simulink model "PGEReducedOrderModel"  (Simulink 8.7)
settings: Solver=ode23tb  StartTime=0.0  StopTime=4  MaxStep=0.04  RelTol=1e-3
undefined symbols (not defined in the file): D1, Delta
libraries: powerlib x98
Description:
  | Copyright 2008-2016 The MathWorks, Inc.
settings Model: Creator=MathWorks  LastModifiedBy=Sayonsom Chanda
settings DataIOCC: SignalLoggingSaveFormat=ModelDataLogs
settings OptimizationCC: ExpressionDepthLimit=2147483647
settings DebuggingCC: SolverPrmCheckMsg=warning  FcnCallInpInsideContextMsg=UseLocalSettings  UnconnectedInputMsg=none  UnconnectedOutputMsg=none  UnconnectedLineMsg=none  StateNameClashWarn=warning
settings GRTTargetCC: CombineOutputUpdateFcns=off  GRTInterface=on
settings ConfigComp: CovSFcnEnable=off

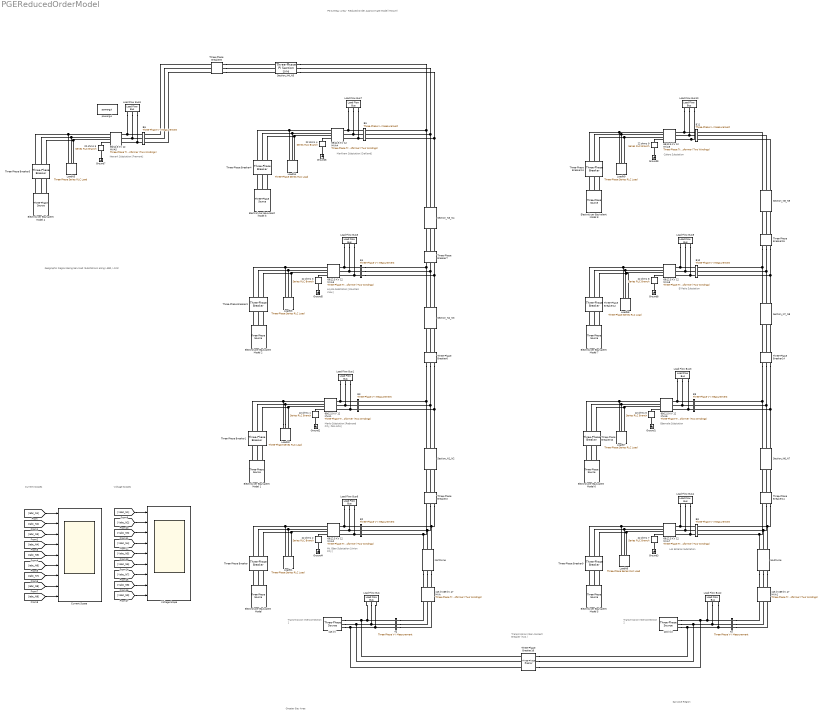
== system PGEReducedOrderModel ==
  note: Geographic Region Being Serviced
      | (Substations along I-880, I-101)
  note: Mt. Eden
      | Substation
      | [Union City]
  note: PG & E Bay Area - Reduced Order Approximate Model (ROAM)
  note: Transmission
      | Interconnection 1
  note: Menlo
      | Substation
      | [Redwood City,
      | Palo Alto]
  note: Loyola
      | Substation
      | [Mountain View]
  note: Markham
      | Substation
      | [Oakland]
  note: Newark
      | Substation
      | [Fremont]
  note: Los Esteros
      | Substation
  note: Transmission
      | Interconnection 2
  note: Edenvale
      | Substation
  note: Calero
      | Substation
  note: Transmission
      | Inter-connect
      | Breaker (N.O.)
  note: Greater Bay Area
  note: San Jose Region
  note: El Patio
      | Substation
  note: Voltage Scopes
  note: Current Scopes
  115 kV : powerlib/Electrical Sources/Three-Phase Source  InternalConnection=Yg  VoltagePhases=off  Voltage=(115000)*1.0445  PhaseAngle=-3.3182  Voltage_phases=[25e3 25e3 25e3]/sqrt(3)  PhaseAngles_phases=[0 -120 +120]  Frequency=60  NonIdealSource=on  SpecifyImpedance=on  Resistance=0.8929  Inductance=16.58e-3  ShortCircuitLevel=2000e6  BaseVoltage=120e3  XRratio=7  BusType=swing  Pref=10000000  Qref=3000000  Prefabc=[10e3, 10e3, 10e3]  Qrefabc=[0, 0, 0]  Qmin=-Inf  Qmax=Inf
  115 kV/69 kV 47 MVA : powerlib/Elements/Three-Phase Transformer (Two Windings)  Winding1Connection=Yg  Winding2Connection=Delta (D1)  CoreType=Three single-phase transformers  SetSaturation=off  Hysteresis=off  DataFile='basic_model'  SetInitialFlux=off  Measurements=None  UNITS=pu  NominalPower=[47e6 60 ]  Winding1="[ 115e3  0.002    0.06 ]"  Winding2="[ 69e3  0.002  0.06]"  Rm=500  Lm=500  L0=0.5  Saturation="[ 0,0  ;  0.005,1.2  ;  1.0,1.4 ]"  InitialFluxes=[ 0.8 , -0.8 , 0.7 ]  MoreParameters=off  BreakLoop=off  DataType=off  TransfoNumber=0
  115 kV/69 kV 47 MVA1 : powerlib/Elements/Three-Phase Transformer (Two Windings)  Winding1Connection=Yg  Winding2Connection=Delta (D1)  CoreType=Three single-phase transformers  SetSaturation=off  Hysteresis=off  DataFile='basic_model'  SetInitialFlux=off  Measurements=None  UNITS=pu  NominalPower=[47e6 60 ]  Winding1="[ 115e3  0.002    0.06 ]"  Winding2="[ 69e3  0.002  0.06]"  Rm=500  Lm=500  L0=0.5  Saturation="[ 0,0  ;  0.005,1.2  ;  1.0,1.4 ]"  InitialFluxes=[ 0.8 , -0.8 , 0.7 ]  MoreParameters=off  BreakLoop=off  DataType=off  TransfoNumber=0
  115 kV2 : powerlib/Electrical Sources/Three-Phase Source  InternalConnection=Yg  VoltagePhases=off  Voltage=(115000)*1.0445  PhaseAngle=-3.3182  Voltage_phases=[25e3 25e3 25e3]/sqrt(3)  PhaseAngles_phases=[0 -120 +120]  Frequency=60  NonIdealSource=on  SpecifyImpedance=on  Resistance=0.8929  Inductance=16.58e-3  ShortCircuitLevel=2000e6  BaseVoltage=115e3  XRratio=7  BusType=swing  Pref=10000000  Qref=3000000  Prefabc=[10e3, 10e3, 10e3]  Qrefabc=[0, 0, 0]  Qmin=-Inf  Qmax=Inf
  22 ohms {1..9} (9 alike) : powerlib/Elements/Series RLC Branch  LConnTagsString=__new0  RConnTagsString=__new0  BranchType=R  Resistance=22  Inductance=1.0  SetiL0=off  InitialCurrent=0  Capacitance=1.0  Setx0=off  InitialVoltage=0  Measurements=None
  69/12.5 KV 12 MVA{1..9} (9 alike) : powerlib/Elements/Three-Phase Transformer (Two Windings)  Winding1Connection=Yg  Winding2Connection=Yn  CoreType=Three single-phase transformers  SetSaturation=off  Hysteresis=off  DataFile='hysteresis'  SetInitialFlux=off  Measurements=None  UNITS=pu  NominalPower="[12e6  60]"  Winding1=[69e3 , 0.025/30 , 0.025]  Winding2=[ 12500, 0.025/30 , 0.025]  Rm=500  Lm=inf  L0=0.5  Saturation=[ 0,0 ; 0.0024,1.2 ; 1.0,1.52 ]  InitialFluxes=[ 0.8 , -0.8 , 0.7 ]  MoreParameters=off  BreakLoop=off  DataType=off  TransfoNumber=0
  B10 : powerlib/Measurements/Three-Phase V-I Measurement  VoltageMeasurement=phase-to-ground  SetLabelV=on  LabelV=Vabc_N8  Vpu=on  VpuLL=off  CurrentMeasurement=yes  SetLabelI=on  LabelI=Iabc_N8  Ipu=on  Pbase=10e6  Vbase=69e3  OutputType=Complex  PhasorSimulation=on  PSBequivalent=0
  B11 : powerlib/Measurements/Three-Phase V-I Measurement  VoltageMeasurement=phase-to-ground  SetLabelV=on  LabelV=Vabc_N9  Vpu=on  VpuLL=off  CurrentMeasurement=yes  SetLabelI=on  LabelI=Iabc_N9  Ipu=on  Pbase=10e6  Vbase=69e3  OutputType=Complex  PhasorSimulation=on  PSBequivalent=0
  B2 : powerlib/Measurements/Three-Phase V-I Measurement  VoltageMeasurement=phase-to-ground  SetLabelV=on  LabelV=Vabc_N1  Vpu=on  VpuLL=off  CurrentMeasurement=yes  SetLabelI=on  LabelI=Iabc_N1  Ipu=on  Pbase=10e6  Vbase=69e3  OutputType=Complex  PhasorSimulation=on  PSBequivalent=0
  B3 : powerlib/Measurements/Three-Phase V-I Measurement  VoltageMeasurement=phase-to-ground  SetLabelV=on  LabelV=Vabc_N2  Vpu=on  VpuLL=off  CurrentMeasurement=yes  SetLabelI=on  LabelI=Iabc_N2  Ipu=on  Pbase=10e6  Vbase=69e3  OutputType=Complex  PhasorSimulation=on  PSBequivalent=0
  B4 : powerlib/Measurements/Three-Phase V-I Measurement  VoltageMeasurement=phase-to-ground  SetLabelV=on  LabelV=Vabc_N3  Vpu=on  VpuLL=off  CurrentMeasurement=yes  SetLabelI=on  LabelI=Iabc_N3  Ipu=on  Pbase=10e6  Vbase=69e3  OutputType=Complex  PhasorSimulation=on  PSBequivalent=0
  B5 : powerlib/Measurements/Three-Phase V-I Measurement  VoltageMeasurement=phase-to-ground  SetLabelV=on  LabelV=Vabc_N4  Vpu=on  VpuLL=off  CurrentMeasurement=yes  SetLabelI=on  LabelI=Iabc_N4  Ipu=on  Pbase=10e6  Vbase=69e3  OutputType=Complex  PhasorSimulation=on  PSBequivalent=0
  B6 : powerlib/Measurements/Three-Phase V-I Measurement  VoltageMeasurement=phase-to-ground  SetLabelV=on  LabelV=Vabc_N5  Vpu=on  VpuLL=off  CurrentMeasurement=yes  SetLabelI=on  LabelI=Iabc_N5  Ipu=on  Pbase=10e6  Vbase=69e3  OutputType=Complex  PhasorSimulation=on  PSBequivalent=0
  B8 : powerlib/Measurements/Three-Phase V-I Measurement  VoltageMeasurement=phase-to-ground  SetLabelV=on  LabelV=Vabc_N6  Vpu=on  VpuLL=off  CurrentMeasurement=yes  SetLabelI=on  LabelI=Iabc_N6  Ipu=on  Pbase=10e6  Vbase=12.5e3  OutputType=Complex  PhasorSimulation=on  PSBequivalent=0
  B9 : powerlib/Measurements/Three-Phase V-I Measurement  VoltageMeasurement=phase-to-ground  SetLabelV=on  LabelV=Vabc_N7  Vpu=on  VpuLL=off  CurrentMeasurement=yes  SetLabelI=on  LabelI=Iabc_N7  Ipu=on  Pbase=10e6  Vbase=69e3  OutputType=Complex  PhasorSimulation=on  PSBequivalent=0
  Current Scope : Scope  NumInputPorts=9
  Electrolyzer Equivalent Model {,2..8} (8 alike) : powerlib/Electrical Sources/Three-Phase Source  InternalConnection=Yg  VoltagePhases=off  Voltage=12.5e3  PhaseAngle=0  Voltage_phases=[25e3 25e3 25e3]/sqrt(3)  PhaseAngles_phases=[0 -120 +120]  Frequency=60  NonIdealSource=on  SpecifyImpedance=off  Resistance=0.8929  Inductance=16.58e-3  ShortCircuitLevel=100e6  BaseVoltage=25e3  XRratio=7  BusType=PQ  Pref=10e3  Qref=0  Prefabc=[10e3, 10e3, 10e3]  Qrefabc=[0, 0, 0]  Qmin=-inf  Qmax=inf
  Electrolyzer Equivalent Model 1 : powerlib/Electrical Sources/Three-Phase Source  InternalConnection=Yg  VoltagePhases=off  Voltage=12.5e3  PhaseAngle=0  Voltage_phases=[25e3 25e3 25e3]/sqrt(3)  PhaseAngles_phases=[0 -120 +120]  Frequency=60  NonIdealSource=on  SpecifyImpedance=off  Resistance=0.8929  Inductance=16.58e-3  ShortCircuitLevel=100e6  BaseVoltage=12.5e3  XRratio=7  BusType=PQ  Pref=10e3  Qref=0  Prefabc=[10e3, 10e3, 10e3]  Qrefabc=[0, 0, 0]  Qmin=-inf  Qmax=inf
  Ground{1..9} (9 alike) : powerlib/Elements/Ground  LConnTagsString=a
  Load Flow Bus : powerlib/Measurements/Load Flow Bus  LConnTagsString=a|b|c  Phases=ABC  Connectors=on one side  ID=T1  Vbase=115e3  Vref=1.02  Vangle=0  VLF=1.02  VLFb=1  VLFc=1  angleLF=0  angleLFb=0  angleLFc=0
      settings: AttributesFormatString=%<ID>\n%<Vbase>V\n%<VLF>pu\n%<angleLF>deg.
  Load Flow Bus1 : powerlib/Measurements/Load Flow Bus  LConnTagsString=a|b|c  Phases=ABC  Connectors=on one side  ID=N2  Vbase=69e3  Vref=1.02  Vangle=0  VLF=1.02  VLFb=1  VLFc=1  angleLF=0  angleLFb=0  angleLFc=0
      settings: AttributesFormatString=%<ID>\n%<Vbase>V\n%<VLF>pu\n%<angleLF>deg.
  Load Flow Bus10 : powerlib/Measurements/Load Flow Bus  LConnTagsString=a|b|c  Phases=ABC  Connectors=on one side  ID=N9  Vbase=69e3  Vref=1.02  Vangle=0  VLF=1.02  VLFb=1  VLFc=1  angleLF=0  angleLFb=0  angleLFc=0
      settings: AttributesFormatString=%<ID>\n%<Vbase>V\n%<VLF>pu\n%<angleLF>deg.
  Load Flow Bus2 : powerlib/Measurements/Load Flow Bus  LConnTagsString=a|b|c  Phases=ABC  Connectors=on one side  ID=T2  Vbase=115e3  Vref=1.02  Vangle=0  VLF=1.02  VLFb=1  VLFc=1  angleLF=0  angleLFb=0  angleLFc=0
      settings: AttributesFormatString=%<ID>\n%<Vbase>V\n%<VLF>pu\n%<angleLF>deg.
  Load Flow Bus3 : powerlib/Measurements/Load Flow Bus  LConnTagsString=a|b|c  Phases=ABC  Connectors=on one side  ID=N7  Vbase=69e3  Vref=1.02  Vangle=0  VLF=1.02  VLFb=1  VLFc=1  angleLF=0  angleLFb=0  angleLFc=0
      settings: AttributesFormatString=%<ID>\n%<Vbase>V\n%<VLF>pu\n%<angleLF>deg.
  Load Flow Bus4 : powerlib/Measurements/Load Flow Bus  LConnTagsString=a|b|c  Phases=ABC  Connectors=on one side  ID=N6  Vbase=69e3  Vref=1.02  Vangle=0  VLF=1.02  VLFb=1  VLFc=1  angleLF=0  angleLFb=0  angleLFc=0
      settings: AttributesFormatString=%<ID>\n%<Vbase>V\n%<VLF>pu\n%<angleLF>deg.
  Load Flow Bus5 : powerlib/Measurements/Load Flow Bus  LConnTagsString=a|b|c  Phases=ABC  Connectors=on one side  ID=N3  Vbase=69e3  Vref=1.02  Vangle=0  VLF=1.02  VLFb=1  VLFc=1  angleLF=0  angleLFb=0  angleLFc=0
      settings: AttributesFormatString=%<ID>\n%<Vbase>V\n%<VLF>pu\n%<angleLF>deg.
  Load Flow Bus6 : powerlib/Measurements/Load Flow Bus  LConnTagsString=a|b|c  Phases=ABC  Connectors=on one side  ID=N1  Vbase=69e3  Vref=1.02  Vangle=0  VLF=1.02  VLFb=1  VLFc=1  angleLF=0  angleLFb=0  angleLFc=0
      settings: AttributesFormatString=%<ID>\n%<Vbase>V\n%<VLF>pu\n%<angleLF>deg.
  Load Flow Bus7 : powerlib/Measurements/Load Flow Bus  LConnTagsString=a|b|c  Phases=ABC  Connectors=on one side  ID=N4  Vbase=69e3  Vref=1.02  Vangle=0  VLF=1.02  VLFb=1  VLFc=1  angleLF=0  angleLFb=0  angleLFc=0
      settings: AttributesFormatString=%<ID>\n%<Vbase>V\n%<VLF>pu\n%<angleLF>deg.
  Load Flow Bus8 : powerlib/Measurements/Load Flow Bus  LConnTagsString=a|b|c  Phases=ABC  Connectors=on one side  ID=N5  Vbase=69e3  Vref=1.02  Vangle=0  VLF=1.02  VLFb=1  VLFc=1  angleLF=0  angleLFb=0  angleLFc=0
      settings: AttributesFormatString=%<ID>\n%<Vbase>V\n%<VLF>pu\n%<angleLF>deg.
  Load Flow Bus9 : powerlib/Measurements/Load Flow Bus  LConnTagsString=a|b|c  Phases=ABC  Connectors=on one side  ID=N8  Vbase=69e3  Vref=1.02  Vangle=0  VLF=1.02  VLFb=1  VLFc=1  angleLF=0  angleLFb=0  angleLFc=0
      settings: AttributesFormatString=%<ID>\n%<Vbase>V\n%<VLF>pu\n%<angleLF>deg.
  LoadN1 : powerlib/Elements/Three-Phase Series RLC Load  LConnTagsString=A|B|C  Configuration=Delta  NominalVoltage=12.5e3  Vabc=[1e3 1e3 1e3]  Vabcp=[1e3 1e3 1e3]  NominalFrequency=60  UnbalancedPower=off  ActivePower=0.89e6/50  InductivePower=0  CapacitivePower=1.2e6  Pabc=[10e3 9e3 11e3]  QLabc=[100 90 110]  QCabc=[100 90 110]  Pabcp=[10e3 9e3 11e3]  QLabcp=[100 90 110]  QCabcp=[100 90 110]  Measurements=None  LoadType=constant PQ
  LoadN{2..9} (8 alike) : powerlib/Elements/Three-Phase Series RLC Load  LConnTagsString=A|B|C  Configuration=Delta  NominalVoltage=12.5e3  Vabc=[1e3 1e3 1e3]  Vabcp=[1e3 1e3 1e3]  NominalFrequency=60  UnbalancedPower=off  ActivePower=1.2e6/50  InductivePower=0  CapacitivePower=1.2e6  Pabc=[10e3 9e3 11e3]  QLabc=[100 90 110]  QCabc=[100 90 110]  Pabcp=[10e3 9e3 11e3]  QLabcp=[100 90 110]  QCabcp=[100 90 110]  Measurements=None  LoadType=constant PQ
  NorthLine : powerlib/Elements/Three-Phase PI Section Line  LConnTagsString=a|b|c  RConnTagsString=A|B|C  Frequency=60  Resistances=[0.1153 0.413]  Inductances=[1.05e-3 3.32e-3]  Capacitances=[11.33e-009 5.01e-009]  Length=25
  Section_N1_N2 : powerlib/Elements/Three-Phase PI Section Line  LConnTagsString=a|b|c  RConnTagsString=A|B|C  Frequency=60  Resistances=[0.1153 0.413]  Inductances=[1.05e-3 3.32e-3]  Capacitances=[11.33e-009 5.01e-009]  Length=25
  Section_N2_N3 : powerlib/Elements/Three-Phase PI Section Line  LConnTagsString=a|b|c  RConnTagsString=A|B|C  Frequency=60  Resistances=[0.1153 0.413]  Inductances=[1.05e-3 3.32e-3]  Capacitances=[11.33e-009 5.01e-009]  Length=25
  Section_N3_N4 : powerlib/Elements/Three-Phase PI Section Line  LConnTagsString=a|b|c  RConnTagsString=A|B|C  Frequency=60  Resistances=[0.1153 0.413]  Inductances=[1.05e-3 3.32e-3]  Capacitances=[11.33e-009 5.01e-009]  Length=25
  Section_N4_N5 : powerlib/Elements/Three-Phase PI Section Line  LConnTagsString=a|b|c  RConnTagsString=A|B|C  Frequency=60  Resistances=[0.1153 0.413]  Inductances=[1.05e-3 3.32e-3]  Capacitances=[11.33e-009 5.01e-009]  Length=25
  Section_N6_N7 : powerlib/Elements/Three-Phase PI Section Line  LConnTagsString=a|b|c  RConnTagsString=A|B|C  Frequency=60  Resistances=[0.1153 0.413]  Inductances=[1.05e-3 3.32e-3]  Capacitances=[11.33e-009 5.01e-009]  Length=25
  Section_N7_N8 : powerlib/Elements/Three-Phase PI Section Line  LConnTagsString=a|b|c  RConnTagsString=A|B|C  Frequency=60  Resistances=[0.1153 0.413]  Inductances=[1.05e-3 3.32e-3]  Capacitances=[11.33e-009 5.01e-009]  Length=25
  Section_N8_N9 : powerlib/Elements/Three-Phase PI Section Line  LConnTagsString=a|b|c  RConnTagsString=A|B|C  Frequency=60  Resistances=[0.1153 0.413]  Inductances=[1.05e-3 3.32e-3]  Capacitances=[11.33e-009 5.01e-009]  Length=25
  SouthLine : powerlib/Elements/Three-Phase PI Section Line  LConnTagsString=a|b|c  RConnTagsString=A|B|C  Frequency=60  Resistances=[0.0153 0.413]  Inductances=[1.05e-3 3.32e-3]  Capacitances=[11.33e-009 5.01e-009]  Length=25
  "T1 " : powerlib/Measurements/Three-Phase V-I Measurement  VoltageMeasurement=phase-to-ground  SetLabelV=on  LabelV=T1  Vpu=on  VpuLL=off  CurrentMeasurement=no  SetLabelI=on  LabelI=Iabc_B120  Ipu=off  Pbase=100e6  Vbase=115e3  OutputType=Complex  PhasorSimulation=on  PSBequivalent=0
  "T2 " : powerlib/Measurements/Three-Phase V-I Measurement  VoltageMeasurement=phase-to-ground  SetLabelV=on  LabelV=T2  Vpu=on  VpuLL=off  CurrentMeasurement=no  SetLabelI=on  LabelI=Iabc_B120  Ipu=off  Pbase=100e6  Vbase=115e3  OutputType=Complex  PhasorSimulation=on  PSBequivalent=0
  Three-Phase Breaker{,1,3..5,9..10,12..13,16} (10 alike) : powerlib/Elements/Three-Phase Breaker  InitialState=open  SwitchA=on  SwitchB=on  SwitchC=on  SwitchTimes="[1/60  5/60]"  External=off  BreakerResistance=0.01  SnubberResistance=1e6  SnubberCapacitance=inf  Measurements=Breaker voltages
  Three-Phase Breaker{2,6..8,11,14..15} (7 alike) : powerlib/Elements/Three-Phase Breaker  InitialState=closed  SwitchA=on  SwitchB=on  SwitchC=on  SwitchTimes="[1/60  5/60]"  External=off  BreakerResistance=0.01  SnubberResistance=1e6  SnubberCapacitance=inf  Measurements=None
  Voltage Scope : Scope  NumInputPorts=9
  powergui : powerlib/powergui  Priority=1  SimulationMode=Phasor  SolverType=Tustin  SampleTime=50e-6  frequency=60  SPID=off  DisableSnubberDevices=off  DisableRonSwitches=off  DisableVfSwitches=off  SwTol=0  DisplayEquations=off  Interpol=off  ExternalGateDelay=off  methode=off  Ts=100  FunctionMessages=off  echomessages=off  HookPort=off  EnableUseOfTLC=off  x0status=blocks  frequencyindice=60  Pbase=100e6  ErrMax=0.0001  Iterations=50  UnitsV=kV  UnitsW=MW  buscounter=0  RestoreLinks=warning  ResistiveCurrentMeasurement=off  Frange=[0:2:500]  Ylog=off  Xlog=on  ShowGrid=off  save=off  variable=ZData  structure=0  ZoomFFT=off  StartTime=0.0  cycles=1  DisplayStyle=1  fundamental=60  FreqAxis=off  MaxFrequency=1000  frequencyindicesteady=1  RmsSteady=1  display=off
  wires:
  [Iabc_N1] -> Current Scope/1
  [Iabc_N2] -> Current Scope/2
  [Iabc_N3] -> Current Scope/3
  [Iabc_N4] -> Current Scope/4
  [Iabc_N5] -> Current Scope/5
  [Iabc_N6] -> Current Scope/6
  [Iabc_N7] -> Current Scope/7
  [Iabc_N8] -> Current Scope/8
  [Iabc_N9] -> Current Scope/9
  [Vabc_N1] -> Voltage Scope/1
  [Vabc_N2] -> Voltage Scope/2
  [Vabc_N3] -> Voltage Scope/3
  [Vabc_N4] -> Voltage Scope/4
  [Vabc_N5] -> Voltage Scope/5
  [Vabc_N6] -> Voltage Scope/6
  [Vabc_N7] -> Voltage Scope/7
  [Vabc_N8] -> Voltage Scope/8
  [Vabc_N9] -> Voltage Scope/9
  connections:
  "T1 "/LConn1 -- Three-Phase Breaker16/RConn1 -- 115 kV/RConn1 -- Load Flow Bus/LConn1
  115 kV/RConn2 -- Three-Phase Breaker16/RConn2 -- Load Flow Bus/LConn2 -- "T1 "/LConn2
  115 kV/RConn3 -- Three-Phase Breaker16/RConn3 -- Load Flow Bus/LConn3 -- "T1 "/LConn3
  "T1 "/RConn1 -- 115 kV/69 kV 47 MVA/RConn3
  "T1 "/RConn2 -- 115 kV/69 kV 47 MVA/RConn2
  "T1 "/RConn3 -- 115 kV/69 kV 47 MVA/RConn1
  NorthLine/LConn3 -- 115 kV/69 kV 47 MVA/LConn1
  NorthLine/LConn2 -- 115 kV/69 kV 47 MVA/LConn2
  NorthLine/LConn1 -- 115 kV/69 kV 47 MVA/LConn3
  NorthLine/RConn1 -- B2/RConn3 -- Three-Phase Breaker2/RConn1
  NorthLine/RConn2 -- Three-Phase Breaker2/RConn2 -- B2/RConn2
  NorthLine/RConn3 -- Three-Phase Breaker2/RConn3 -- B2/RConn1
  B2/LConn1 -- Load Flow Bus6/LConn1 -- 69/12.5 KV 12 MVA2/LConn1
  B2/LConn2 -- Load Flow Bus6/LConn2 -- 69/12.5 KV 12 MVA2/LConn2
  B2/LConn3 -- Load Flow Bus6/LConn3 -- 69/12.5 KV 12 MVA2/LConn3
  Ground4/LConn1 -- 22 ohms 2/RConn1
  69/12.5 KV 12 MVA2/RConn4 -- 22 ohms 2/LConn1
  69/12.5 KV 12 MVA2/RConn3 -- LoadN1/LConn3 -- Three-Phase Breaker/LConn3
  69/12.5 KV 12 MVA2/RConn2 -- LoadN1/LConn2 -- Three-Phase Breaker/LConn2
  69/12.5 KV 12 MVA2/RConn1 -- LoadN1/LConn1 -- Three-Phase Breaker/LConn1
  "Electrolyzer Equivalent Model "/RConn3 -- Three-Phase Breaker/RConn3
  "Electrolyzer Equivalent Model "/RConn2 -- Three-Phase Breaker/RConn2
  "Electrolyzer Equivalent Model "/RConn1 -- Three-Phase Breaker/RConn1
  Section_N1_N2/RConn3 -- Three-Phase Breaker6/RConn3 -- B3/RConn3
  Section_N1_N2/RConn2 -- B3/RConn2 -- Three-Phase Breaker6/RConn2
  Section_N1_N2/RConn1 -- Three-Phase Breaker6/RConn1 -- B3/RConn1
  B3/LConn1 -- Load Flow Bus1/LConn1 -- 69/12.5 KV 12 MVA1/LConn1
  B3/LConn2 -- Load Flow Bus1/LConn2 -- 69/12.5 KV 12 MVA1/LConn2
  B3/LConn3 -- Load Flow Bus1/LConn3 -- 69/12.5 KV 12 MVA1/LConn3
  69/12.5 KV 12 MVA1/RConn3 -- Three-Phase Breaker1/LConn3 -- LoadN2/LConn3
  LoadN2/LConn2 -- 69/12.5 KV 12 MVA1/RConn2 -- Three-Phase Breaker1/LConn2
  LoadN2/LConn1 -- 69/12.5 KV 12 MVA1/RConn1 -- Three-Phase Breaker1/LConn1
  Electrolyzer Equivalent Model 1/RConn3 -- Three-Phase Breaker1/RConn3
  Ground2/LConn1 -- 22 ohms 1/RConn1
  Electrolyzer Equivalent Model 1/RConn2 -- Three-Phase Breaker1/RConn2
  69/12.5 KV 12 MVA1/RConn4 -- 22 ohms 1/LConn1
  Electrolyzer Equivalent Model 1/RConn1 -- Three-Phase Breaker1/RConn1
  Three-Phase Breaker2/LConn3 -- Section_N1_N2/LConn3
  Three-Phase Breaker2/LConn2 -- Section_N1_N2/LConn2
  Three-Phase Breaker2/LConn1 -- Section_N1_N2/LConn1
  B4/LConn1 -- Load Flow Bus5/LConn1 -- 69/12.5 KV 12 MVA3/LConn1
  B4/LConn2 -- Load Flow Bus5/LConn2 -- 69/12.5 KV 12 MVA3/LConn2
  B4/LConn3 -- Load Flow Bus5/LConn3 -- 69/12.5 KV 12 MVA3/LConn3
  69/12.5 KV 12 MVA3/RConn3 -- LoadN3/LConn3 -- Three-Phase Breaker3/LConn3
  69/12.5 KV 12 MVA3/RConn2 -- LoadN3/LConn2 -- Three-Phase Breaker3/LConn2
  69/12.5 KV 12 MVA3/RConn1 -- LoadN3/LConn1 -- Three-Phase Breaker3/LConn1
  Electrolyzer Equivalent Model 2/RConn1 -- Three-Phase Breaker3/RConn1
  Ground5/LConn1 -- 22 ohms 3/RConn1
  69/12.5 KV 12 MVA3/RConn4 -- 22 ohms 3/LConn1
  Electrolyzer Equivalent Model 2/RConn2 -- Three-Phase Breaker3/RConn2
  Electrolyzer Equivalent Model 2/RConn3 -- Three-Phase Breaker3/RConn3
  B5/LConn1 -- Load Flow Bus7/LConn1 -- 69/12.5 KV 12 MVA4/LConn1
  B5/LConn2 -- Load Flow Bus7/LConn2 -- 69/12.5 KV 12 MVA4/LConn2
  B5/LConn3 -- Load Flow Bus7/LConn3 -- 69/12.5 KV 12 MVA4/LConn3
  69/12.5 KV 12 MVA4/RConn3 -- LoadN4/LConn3 -- Three-Phase Breaker4/LConn3
  69/12.5 KV 12 MVA4/RConn2 -- LoadN4/LConn2 -- Three-Phase Breaker4/LConn2
  69/12.5 KV 12 MVA4/RConn1 -- LoadN4/LConn1 -- Three-Phase Breaker4/LConn1
  Electrolyzer Equivalent Model 3/RConn3 -- Three-Phase Breaker4/RConn3
  Electrolyzer Equivalent Model 3/RConn1 -- Three-Phase Breaker4/RConn1
  Ground6/LConn1 -- 22 ohms 4/RConn1
  Section_N3_N4/RConn1 -- Section_N4_N5/RConn1 -- B5/RConn1
  Electrolyzer Equivalent Model 3/RConn2 -- Three-Phase Breaker4/RConn2
  Section_N3_N4/RConn2 -- Section_N4_N5/RConn2 -- B5/RConn2
  Section_N3_N4/RConn3 -- Section_N4_N5/RConn3 -- B5/RConn3
  69/12.5 KV 12 MVA4/RConn4 -- 22 ohms 4/LConn1
  B6/LConn1 -- Load Flow Bus8/LConn1 -- 69/12.5 KV 12 MVA5/LConn1
  B6/LConn2 -- Load Flow Bus8/LConn2 -- 69/12.5 KV 12 MVA5/LConn2
  B6/LConn3 -- Load Flow Bus8/LConn3 -- 69/12.5 KV 12 MVA5/LConn3
  69/12.5 KV 12 MVA5/RConn3 -- LoadN5/LConn3 -- Three-Phase Breaker5/LConn3
  69/12.5 KV 12 MVA5/RConn2 -- LoadN5/LConn2 -- Three-Phase Breaker5/LConn2
  69/12.5 KV 12 MVA5/RConn1 -- LoadN5/LConn1 -- Three-Phase Breaker5/LConn1
  Electrolyzer Equivalent Model 4/RConn3 -- Three-Phase Breaker5/RConn3
  Electrolyzer Equivalent Model 4/RConn1 -- Three-Phase Breaker5/RConn1
  Ground7/LConn1 -- 22 ohms 5/RConn1
  Three-Phase Breaker8/RConn1 -- B6/RConn1
  Electrolyzer Equivalent Model 4/RConn2 -- Three-Phase Breaker5/RConn2
  Three-Phase Breaker8/RConn2 -- B6/RConn2
  Three-Phase Breaker8/RConn3 -- B6/RConn3
  69/12.5 KV 12 MVA5/RConn4 -- 22 ohms 5/LConn1
  Three-Phase Breaker6/LConn2 -- Section_N2_N3/LConn2
  Three-Phase Breaker6/LConn1 -- Section_N2_N3/LConn1
  Three-Phase Breaker6/LConn3 -- Section_N2_N3/LConn3
  Three-Phase Breaker7/LConn2 -- Section_N3_N4/LConn2
  Three-Phase Breaker7/LConn1 -- Section_N3_N4/LConn1
  Three-Phase Breaker7/LConn3 -- Section_N3_N4/LConn3
  Three-Phase Breaker8/LConn2 -- Section_N4_N5/LConn2
  Three-Phase Breaker8/LConn1 -- Section_N4_N5/LConn1
  Three-Phase Breaker8/LConn3 -- Section_N4_N5/LConn3
  Load Flow Bus2/LConn1 -- Three-Phase Breaker16/LConn3 -- 115 kV2/RConn1 -- "T2 "/LConn1
  115 kV2/RConn2 -- Three-Phase Breaker16/LConn2 -- Load Flow Bus2/LConn2 -- "T2 "/LConn2
  115 kV2/RConn3 -- Three-Phase Breaker16/LConn1 -- "T2 "/LConn3 -- Load Flow Bus2/LConn3
  Three-Phase Breaker11/RConn1 -- SouthLine/RConn1 -- B8/RConn3
  Three-Phase Breaker11/RConn2 -- SouthLine/RConn2 -- B8/RConn2
  SouthLine/RConn3 -- Three-Phase Breaker11/RConn3 -- B8/RConn1
  B8/LConn1 -- Load Flow Bus4/LConn1 -- 69/12.5 KV 12 MVA7/LConn1
  B8/LConn2 -- Load Flow Bus4/LConn2 -- 69/12.5 KV 12 MVA7/LConn2
  B8/LConn3 -- Load Flow Bus4/LConn3 -- 69/12.5 KV 12 MVA7/LConn3
  69/12.5 KV 12 MVA7/RConn3 -- LoadN6/LConn3 -- Three-Phase Breaker9/LConn3
  69/12.5 KV 12 MVA7/RConn2 -- LoadN6/LConn2 -- Three-Phase Breaker9/LConn2
  69/12.5 KV 12 MVA7/RConn1 -- LoadN6/LConn1 -- Three-Phase Breaker9/LConn1
  Section_N6_N7/RConn3 -- Three-Phase Breaker14/RConn3 -- B9/RConn3
  Section_N6_N7/RConn2 -- Three-Phase Breaker14/RConn2 -- B9/RConn2
  Section_N6_N7/RConn1 -- Three-Phase Breaker14/RConn1 -- B9/RConn1
  B9/LConn1 -- Load Flow Bus3/LConn1 -- 69/12.5 KV 12 MVA6/LConn1
  B9/LConn2 -- Load Flow Bus3/LConn2 -- 69/12.5 KV 12 MVA6/LConn2
  B9/LConn3 -- Load Flow Bus3/LConn3 -- 69/12.5 KV 12 MVA6/LConn3
  69/12.5 KV 12 MVA6/RConn3 -- LoadN7/LConn3 -- Three-Phase Breaker10/LConn3
  69/12.5 KV 12 MVA6/RConn2 -- LoadN7/LConn2 -- Three-Phase Breaker10/LConn2
  69/12.5 KV 12 MVA6/RConn1 -- LoadN7/LConn1 -- Three-Phase Breaker10/LConn1
  B10/LConn1 -- Load Flow Bus9/LConn1 -- 69/12.5 KV 12 MVA8/LConn1
  B10/LConn2 -- Load Flow Bus9/LConn2 -- 69/12.5 KV 12 MVA8/LConn2
  B10/LConn3 -- Load Flow Bus9/LConn3 -- 69/12.5 KV 12 MVA8/LConn3
  69/12.5 KV 12 MVA8/RConn3 -- LoadN8/LConn3 -- Three-Phase Breaker12/LConn3
  69/12.5 KV 12 MVA8/RConn2 -- Three-Phase Breaker12/LConn2 -- LoadN8/LConn2
  69/12.5 KV 12 MVA8/RConn1 -- Three-Phase Breaker12/LConn1 -- LoadN8/LConn1
  B11/LConn1 -- 69/12.5 KV 12 MVA9/LConn1 -- Load Flow Bus10/LConn1
  B11/LConn2 -- 69/12.5 KV 12 MVA9/LConn2 -- Load Flow Bus10/LConn2
  B11/LConn3 -- 69/12.5 KV 12 MVA9/LConn3 -- Load Flow Bus10/LConn3
  Three-Phase Breaker11/LConn1 -- Section_N6_N7/LConn1
  Three-Phase Breaker15/LConn3 -- Section_N8_N9/LConn3
  Ground3/LConn1 -- 22 ohms 7/RConn1
  69/12.5 KV 12 MVA7/RConn4 -- 22 ohms 7/LConn1
  Electrolyzer Equivalent Model 8/RConn3 -- Three-Phase Breaker13/RConn3
  Electrolyzer Equivalent Model 6/RConn2 -- Three-Phase Breaker10/RConn2
  Electrolyzer Equivalent Model 6/RConn1 -- Three-Phase Breaker10/RConn1
  Electrolyzer Equivalent Model 8/RConn1 -- Three-Phase Breaker13/RConn1
  Ground9/LConn1 -- 22 ohms 9/RConn1
  Three-Phase Breaker15/LConn1 -- Section_N8_N9/LConn1
  Electrolyzer Equivalent Model 5/RConn1 -- Three-Phase Breaker9/RConn1
  SouthLine/LConn1 -- 115 kV/69 kV 47 MVA1/LConn3
  Section_N8_N9/RConn1 -- B11/RConn1
  Section_N8_N9/RConn3 -- B11/RConn3
  Three-Phase Breaker11/LConn3 -- Section_N6_N7/LConn3
  69/12.5 KV 12 MVA6/RConn4 -- 22 ohms 6/LConn1
  Ground1/LConn1 -- 22 ohms 6/RConn1
  Electrolyzer Equivalent Model 7/RConn3 -- Three-Phase Breaker12/RConn3
  "T2 "/RConn1 -- 115 kV/69 kV 47 MVA1/RConn3
  Ground8/LConn1 -- 22 ohms 8/RConn1
  Section_N7_N8/RConn3 -- Three-Phase Breaker15/RConn3 -- B10/RConn3
  Three-Phase Breaker14/LConn3 -- Section_N7_N8/LConn3
  Electrolyzer Equivalent Model 5/RConn3 -- Three-Phase Breaker9/RConn3
  69/12.5 KV 12 MVA9/RConn4 -- 22 ohms 9/LConn1
  Electrolyzer Equivalent Model 7/RConn2 -- Three-Phase Breaker12/RConn2
  Section_N7_N8/RConn2 -- Three-Phase Breaker15/RConn2 -- B10/RConn2
  Section_N7_N8/RConn1 -- Three-Phase Breaker15/RConn1 -- B10/RConn1
  69/12.5 KV 12 MVA8/RConn4 -- 22 ohms 8/LConn1
  Three-Phase Breaker15/LConn2 -- Section_N8_N9/LConn2
  Three-Phase Breaker14/LConn1 -- Section_N7_N8/LConn1
  Electrolyzer Equivalent Model 5/RConn2 -- Three-Phase Breaker9/RConn2
  SouthLine/LConn2 -- 115 kV/69 kV 47 MVA1/LConn2
  Electrolyzer Equivalent Model 7/RConn1 -- Three-Phase Breaker12/RConn1
  "T2 "/RConn3 -- 115 kV/69 kV 47 MVA1/RConn1
  "T2 "/RConn2 -- 115 kV/69 kV 47 MVA1/RConn2
  Electrolyzer Equivalent Model 8/RConn2 -- Three-Phase Breaker13/RConn2
  SouthLine/LConn3 -- 115 kV/69 kV 47 MVA1/LConn1
  Three-Phase Breaker14/LConn2 -- Section_N7_N8/LConn2
  Three-Phase Breaker11/LConn2 -- Section_N6_N7/LConn2
  Section_N8_N9/RConn2 -- B11/RConn2
  Electrolyzer Equivalent Model 6/RConn3 -- Three-Phase Breaker10/RConn3
  Section_N2_N3/RConn3 -- B4/RConn3 -- Three-Phase Breaker7/RConn3
  Section_N2_N3/RConn2 -- B4/RConn2 -- Three-Phase Breaker7/RConn2
  Section_N2_N3/RConn1 -- B4/RConn1 -- Three-Phase Breaker7/RConn1
  69/12.5 KV 12 MVA9/RConn3 -- Three-Phase Breaker13/LConn3 -- LoadN9/LConn3
  69/12.5 KV 12 MVA9/RConn2 -- Three-Phase Breaker13/LConn2 -- LoadN9/LConn2
  69/12.5 KV 12 MVA9/RConn1 -- Three-Phase Breaker13/LConn1 -- LoadN9/LConn1
